simulink model "sl_subsys_overview"  (Simulink 7.6)
settings: Solver=ode45  StartTime=0.0  StopTime=10.0  RelTol=1e-3
Description:
  | Types of subsystem hierarchies
  | 
  | Simulink consists of two classes of subsystems:
  | 
  | 1) Virtual subsystems: provide graphical hierarchy in models. Virtual
  |    subsystems do not impact model execution. During model execution, the
  |    Simulink Engine flattens all virtual subsystems.
  | 
  | 2) Nonvirtual subsystems: provide execution and graphical hierarchy in models.
  |    Nonvirtual subsystems are executed as a single unit (atomic execution) by
  |    the Simulink Engine. All nonvirtual subsystems are drawn with a bold border.
settings Model: Creator=The MathWorks Inc.  CovMetricSettings=d  ExtModeAutoUpdateStatusClock=off  BufferReuse=off
settings DataIOCC: SignalLoggingName=logsOut
settings OptimizationCC: BlockReduction=off  BooleanDataType=off  InlineInvariantSignals=on  OptimizeBlockIOStorage=off  BufferReuse=off  ExpressionFolding=off  LocalBlockOutputs=off  InitFltsAndDblsToZero=on
settings DebuggingCC: SaveWithParameterizedLinksMsg=none  CheckExecutionContextPreStartOutputMsg=on  CheckExecutionContextRuntimeOutputMsg=on  SignalResolutionControl=TryResolveAllWithWarning  SolverPrmCheckMsg=none  MultiTaskDSMMsg=warning  MultiTaskCondExecSysMsg=none
settings HardwareCC: ProdHWDeviceType=Specified
settings ModelReferenceCC: UpdateModelReferenceTargets=IfOutOfDate
settings RTWCC: IncludeERTFirstTime=on
settings CodeAppCC: CustomSymbolStrFcn=$F$N$M
settings GRTTargetCC: TargetFcnLib=ansi_tfl_tmw.mat

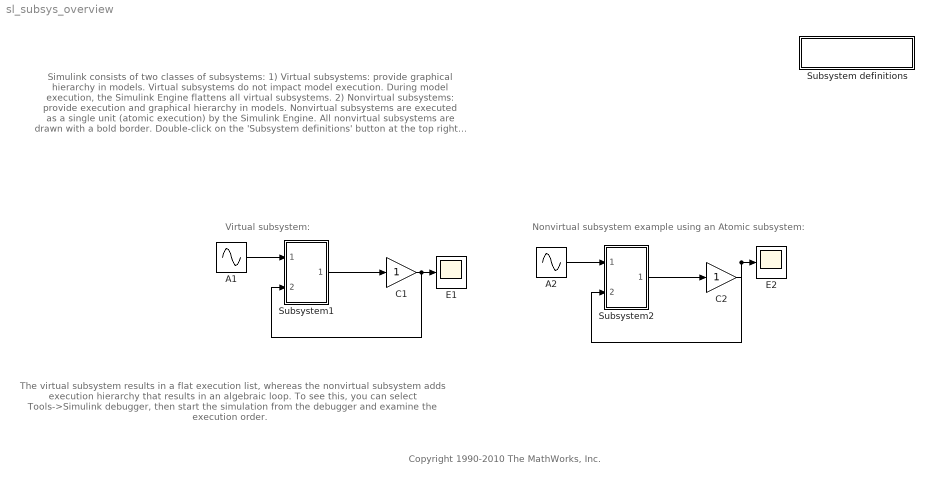
== system sl_subsys_overview ==
  note: Simulink consists of two classes of subsystems:
      |
      | 1) Virtual subsystems: provide graphical hierarchy in models. Virtual
      |    subsystems do not impact model execution. During model execution, the
      |    Simulink Engine flattens all virtual subsystems.
      |
      | 2) Nonvirtual subsystems: provide execution and graphical hierarchy in models.
      |    Nonvirtual subsystems are executed as a single unit (atomic execution) by
      |    the Simulink Engine. All nonvirtual subsystems are drawn with a bold border.
      |
      | Double-click on the 'Subsystem definitions' button at the top right for more details.
  note: Nonvirtual subsystem example using an Atomic subsystem:
  note: Virtual subsystem:
  note: The virtual subsystem results in a flat execution list, whereas the nonvirtual subsystem
      | adds execution hierarchy that results in an algebraic loop. To see this, you can select
      | Tools->Simulink debugger, then start the simulation from the debugger and examine
      |  the execution order.
  note: Copyright 1990-2010 The MathWorks, Inc.
  " Subsystem definitions" : Subsystem
      settings: OpenFcn=helpview([matlabroot,'/toolbox/simulink/simdemos/simfeatures/html/sl_subsys_definitions.html']);
      mask Display: disp('Subsystem\ndefinitions')
  A1 : Sin  SampleTime=0
  A2 : Sin  SampleTime=0
  C1 : Gain  SaturateOnIntegerOverflow=on  OutDataTypeStr=Inherit: Same as input  ParamDataTypeStr=Inherit: Same as input
  C2 : Gain  SaturateOnIntegerOverflow=on  OutDataTypeStr=Inherit: Same as input  ParamDataTypeStr=Inherit: Same as input
  E1 : Scope
  E2 : Scope
  Subsystem1 : Subsystem
  Subsystem2 : Subsystem  TreatAsAtomicUnit=on
  wires:
  A1/1 -> Subsystem1/1(In1)
  Subsystem1/1(Out1) -> C1/1
  C1/1 -> Subsystem1/2(In2), E1/1
  A2/1 -> Subsystem2/1(In1)
  Subsystem2/1(Out1) -> C2/1
  C2/1 -> E2/1, Subsystem2/2(In2)

== system sl_subsys_overview/ Subsystem definitions ==

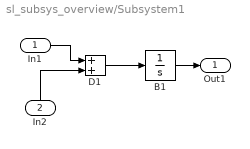
== system sl_subsys_overview/Subsystem1 ==
  In1 : Inport
  In2 : Inport  Port=2
  B1 : Integrator
  D1 : Sum  SaturateOnIntegerOverflow=on  InputSameDT=on  OutDataTypeStr=Inherit: Same as first input
  Out1 : Outport
  wires:
  In1/1 -> D1/1
  B1/1 -> Out1/1
  In2/1 -> D1/2
  D1/1 -> B1/1

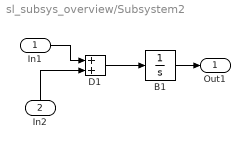
== system sl_subsys_overview/Subsystem2 ==
  In1 : Inport
  In2 : Inport  Port=2
  B1 : Integrator
  D1 : Sum  SaturateOnIntegerOverflow=on  InputSameDT=on  OutDataTypeStr=Inherit: Same as first input
  Out1 : Outport
  wires:
  D1/1 -> B1/1
  In2/1 -> D1/2
  B1/1 -> Out1/1
  In1/1 -> D1/1
